simulink model "simulation"  (R2022b)
settings: Solver=ode45  StartTime=0.0  StopTime=463  RelTol=1e-3  EnableMultiTasking=on
settings Model: Creator=think  LastModifiedBy=linhao
settings SolverCC: AlgebraicLoopSolver=TrustRegion
settings DataIOCC: LimitDataPoints=on  SaveFormat=Array  ReturnWorkspaceOutputs=off
settings OptimizationCC: LifeSpan=inf
settings DebuggingCC: SolverPrmCheckMsg=warning  UnconnectedInputMsg=warning  UnconnectedOutputMsg=warning  UnconnectedLineMsg=warning  SFUnexpectedBacktrackingDiag=warning  SFNoUnconditionalDefaultTransitionDiag=warning  SFExecutionAtInitializationDiag=none  SFMachineParentedDataDiag=warning  ArithmeticOperatorsInVariantConditions=warning
settings HardwareCC: ProdBitPerPointer=32  ProdBitPerSizeT=32  ProdBitPerPtrDiffT=32  ProdLargestAtomicFloat=None  ProdIntDivRoundTo=Undefined  ProdEndianess=Unspecified  ProdWordSize=32  ProdHWDeviceType=32-bit Generic
settings ModelReferenceCC: EnableRefExpFcnMdlSchedulingChecks=on  PropagateSignalLabelsOutOfModel=off
settings SFSimCC: SimUseLocalCustomCode=off  CustomCodeUndefinedFunction=UseInterfaceOnly
settings RTWCC: RTWUseLocalCustomCode=off
settings CodeAppCC: StateflowObjectComments=on
settings GRTTargetCC: TargetLangStandard=C89/C90 (ANSI)
settings ConfigComp: CovMetricSettings=dw  CovSaveCumulativeToWorkspaceVar=on  CovSaveSingleToWorkspaceVar=on  CovExternalEMLEnable=off  CovSFcnEnable=off

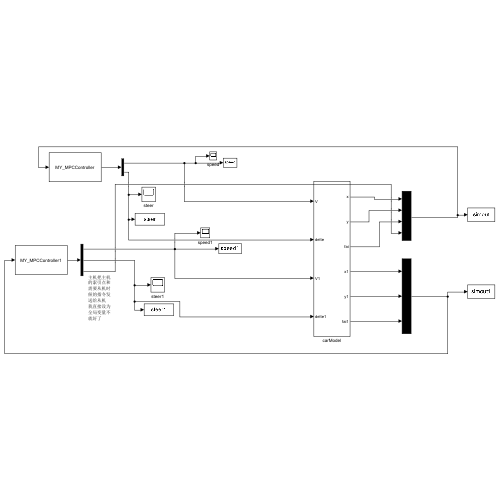
[thumbnail: Simulink's stored preview of the top-level diagram]
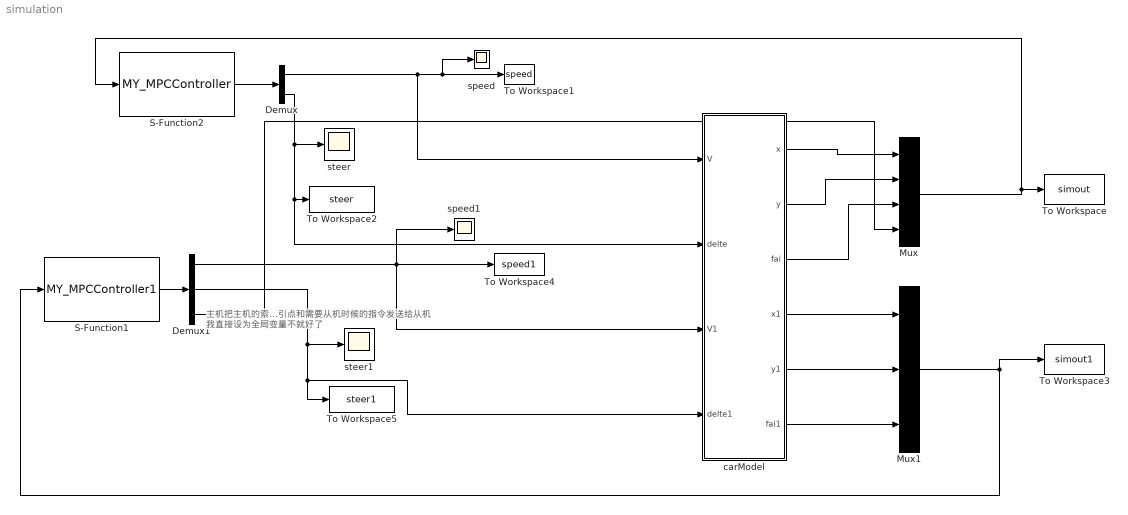
== system simulation ==
  note: 主机把主机的索引点和需要从机时候的指令发送给从机
      | 我直接设为全局变量不就好了
  Demux : Demux  Outputs=2
  Demux1 : Demux  Outputs=3
  Mux : Mux
  Mux1 : Mux  Inputs=3
  S-Function1 : S-Function  FunctionName=MY_MPCController1  SFunctionDeploymentMode=off  EnableBusSupport=off
  S-Function2 : S-Function  FunctionName=MY_MPCController  SFunctionDeploymentMode=off  EnableBusSupport=off
  To Workspace : ToWorkspace  VariableName=simout  SaveFormat=Timeseries  SampleTime=-1
  To Workspace1 : ToWorkspace  VariableName=speed  SaveFormat=Timeseries  SampleTime=-1
  To Workspace2 : ToWorkspace  VariableName=steer  SaveFormat=Timeseries  SampleTime=-1
  To Workspace3 : ToWorkspace  VariableName=simout1  SaveFormat=Timeseries  SampleTime=-1
  To Workspace4 : ToWorkspace  VariableName=speed1  SaveFormat=Timeseries  SampleTime=-1
  To Workspace5 : ToWorkspace  VariableName=steer1  SaveFormat=Timeseries  SampleTime=-1
  carModel : Subsystem
  speed : Scope
  speed1 : Scope
  steer : Scope
  steer1 : Scope
  wires:
  carModel/1(x) -> Mux/1
  Demux1/2 -> To Workspace5/1, carModel/4(delte1), steer1/1
  Demux/1 -> carModel/1(V), To Workspace1/1, speed/1
  carModel/2(y) -> Mux/2
  S-Function1/1 -> Demux1/1
  Demux/2 -> carModel/2(delte), To Workspace2/1, steer/1
  Demux1/1 -> carModel/3(V1), To Workspace4/1, speed1/1
  carModel/5(y1) -> Mux1/2
  Mux/1 -> S-Function2/1, To Workspace/1
  S-Function2/1 -> Demux/1
  carModel/6(fai1) -> Mux1/3
  Mux1/1 -> S-Function1/1, To Workspace3/1
  carModel/4(x1) -> Mux1/1
  Demux1/3 -> Mux/4
  carModel/3(fai) -> Mux/3

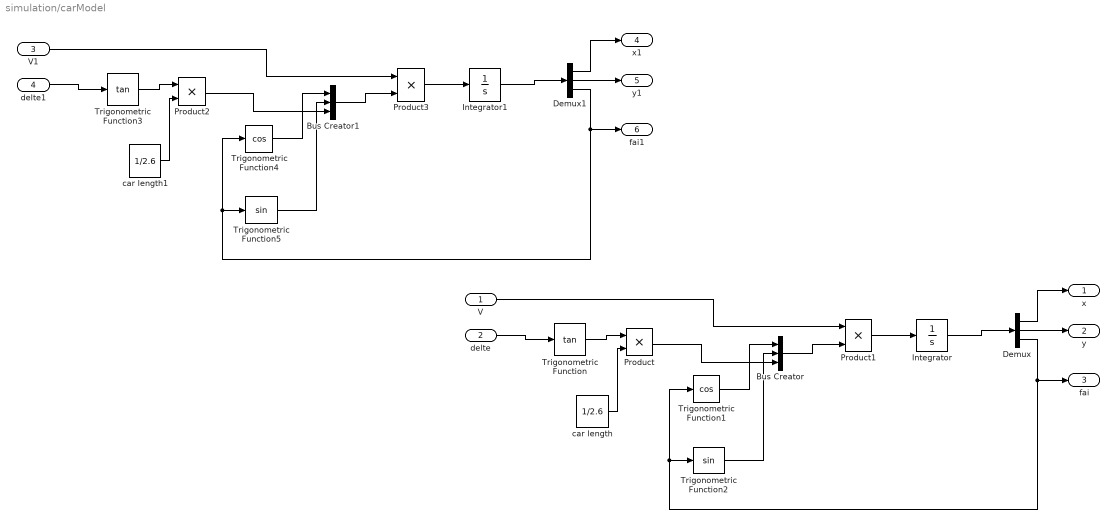
== system simulation/carModel ==
  V : Inport
  delte : Inport  Port=2
  V1 : Inport  Port=3
  delte1 : Inport  Port=4
  Bus Creator : BusCreator  Inputs=3
  Bus Creator1 : BusCreator  Inputs=3
  Demux : Demux  Outputs=3
  Demux1 : Demux  Outputs=3
  Integrator : Integrator  InitialCondition=[0 -8 0]
  Integrator1 : Integrator  InitialCondition=[0 -4 0]
  Product{,1..3} (4 alike) : Product
  Trigonometric Function : Trigonometry  Operator=tan
  Trigonometric Function1 : Trigonometry  Operator=cos
  Trigonometric Function2 : Trigonometry
  Trigonometric Function3 : Trigonometry  Operator=tan
  Trigonometric Function4 : Trigonometry  Operator=cos
  Trigonometric Function5 : Trigonometry
  car length : Constant  Value=1/2.6
  car length1 : Constant  Value=1/2.6
  x : Outport
  y : Outport  Port=2
  fai : Outport  Port=3
  x1 : Outport  Port=4
  y1 : Outport  Port=5
  fai1 : Outport  Port=6
  wires:
  delte/1 -> Trigonometric Function/1
  Bus Creator/1 -> Product1/2
  Product1/1 -> Integrator/1
  Demux/2 -> y/1
  Demux/3 -> Trigonometric Function1/1, Trigonometric Function2/1, fai/1
  car length/1 -> Product/2
  Trigonometric Function/1 -> Product/1
  Demux/1 -> x/1
  Integrator/1 -> Demux/1
  Trigonometric Function1/1 -> Bus Creator/1
  Trigonometric Function2/1 -> Bus Creator/2
  Product/1 -> Bus Creator/3
  V/1 -> Product1/1
  Trigonometric Function4/1 -> Bus Creator1/1
  Product2/1 -> Bus Creator1/3
  V1/1 -> Product3/1
  Product3/1 -> Integrator1/1
  Integrator1/1 -> Demux1/1
  Trigonometric Function5/1 -> Bus Creator1/2
  car length1/1 -> Product2/2
  Demux1/2 -> y1/1
  Demux1/3 -> Trigonometric Function4/1, Trigonometric Function5/1, fai1/1
  delte1/1 -> Trigonometric Function3/1
  Bus Creator1/1 -> Product3/2
  Trigonometric Function3/1 -> Product2/1
  Demux1/1 -> x1/1
